simulink model "simexa22"  (Simulink 2.09)
settings: Solver=ode45  StartTime=0.0  StopTime=3  MaxStep=0.01  RelTol=1e-3  AbsTol=1e-3
settings Model: SaveTime=off  SaveOutput=off  ConsistencyChecking=off  RTWTemplateMakefile=grt_vc.tmf

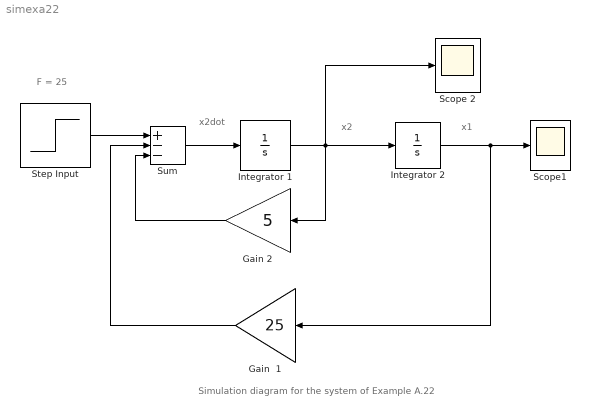
== system simexa22 ==
  note: x1
  note: x2
  note: x2dot
  note: F = 25
  note: Simulation diagram for the system of Example A.22
  Gain  1 : Gain  Orientation=left  Gain=25
  Gain 2 : Gain  Orientation=left  Gain=5
  Integrator 1 : Integrator  ExternalReset=none  InitialConditionSource=internal  InitialCondition=0  LimitOutput=off  UpperSaturationLimit=inf  LowerSaturationLimit=-inf  ShowSaturationPort=off  ShowStatePort=off  AbsoluteTolerance=auto
  Integrator 2 : Integrator  ExternalReset=none  InitialConditionSource=internal  InitialCondition=0  LimitOutput=off  UpperSaturationLimit=inf  LowerSaturationLimit=-inf  ShowSaturationPort=off  ShowStatePort=off  AbsoluteTolerance=auto
  Scope 2 : Scope
      settings: TickLabels=on  TimeRange=auto  YMin=-5  YMax=5  SaveToWorkspace=off  SaveName=ScopeData
  Scope1 : Scope
      settings: TickLabels=on  TimeRange=auto  YMin=-5  YMax=5  SaveToWorkspace=off  SaveName=ScopeData
  Step Input : Step  Time=100  Before=25  After=25
  Sum : Sum  Inputs=+--
  wires:
  Step Input/1 -> Sum/1
  Sum/1 -> Integrator 1/1
  Gain 2/1 -> Sum/3
  Integrator 2/1 -> Scope1/1, Gain  1/1
  Gain  1/1 -> Sum/2
  Integrator 1/1 -> Integrator 2/1, Scope 2/1, Gain 2/1
